simulink model "BidirectionalConverterBuckBoost"  (R2024a)
settings: Solver=VariableStepAuto  StartTime=0.0  StopTime=0.5  MaxStep=1e-6  RelTol=1e-3
undefined symbols (not defined in the file or in its folder): Ion, Lithium
libraries: spsSeriesRLCBranchLib x7, spsCurrentMeasurementLib x3, spsMosfetLib x2, spsVoltageMeasurementLib x2, spsBatteryLib x1, spsPVArrayLib x1, spsPWMGeneratorDCDCLib x1, SignalEditorBlockLib x1, sps_lib x1
settings Model: Creator=Owner  LastModifiedBy=Akbar
settings SolverCC: AlgebraicLoopSolver=TrustRegion
settings DebuggingCC: UnconnectedInputMsg=warning  UnconnectedOutputMsg=warning  UnconnectedLineMsg=warning
settings ModelReferenceCC: EnableRefExpFcnMdlSchedulingChecks=on
settings RTWCC: GPUComputeCapability=3.5

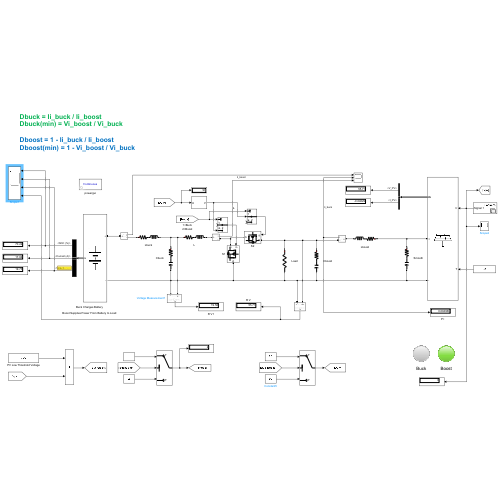
[thumbnail: Simulink's stored preview of the top-level diagram]
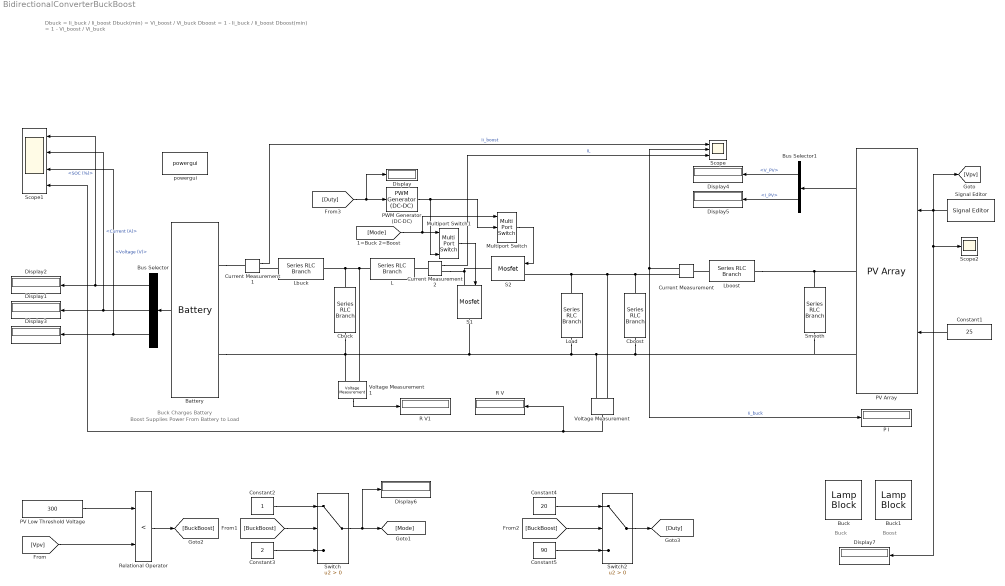
== system BidirectionalConverterBuckBoost ==
  note: Buck
  note: Buck Charges Battery
  note: Dbuck = Ii_buck / Ii_boost
      | Dbuck(min) = Vi_boost / Vi_buck
      |
      | Dboost = 1 - Ii_buck / Ii_boost
      | Dboost(min) = 1 - Vi_boost / Vi_buck
  note: Boost Supplies Power From Battery to Load
  note: Boost
  Battery : spsBatteryLib/Battery  BatType=Lithium-Ion  ShowTempParam=off  ThermalPreset=no  ShowAgeParam=off  NomV=25  NomQ=0.5  SOC=70  Batt_Tr=1  PresetModel=on  MaxQ=0.5  MinV=18.75  FullV=29.0997  Dis_rate=0.21739  R=0.5  Normal_OP=0.45217  expZone="[27.0096    0.0245652]"  current=[6.5 13 32.5]  Units=Time  Tci=20  NomT=20  T2=-30  MaxQ2=4.8  FullV2=7.1  Normal_OP2=5.655  expZone2="[6.58           1]"  Rca=0.6  ti=2000  Dp=0  Neq0=0  Tsim=1e6  Ta1=25  Qeol=5.4*0.9  Reol=0.013333*1.2  Char_age=[2.3478, 3]  Dis_age=[2.3478, 10]  N1=1500  N2=10500  N3=1000  N4=1400  Ta2=45  N5=950
  Buck : LampBlock  LabelPosition=Hide
  Buck1 : LampBlock  LabelPosition=Hide
  Bus Selector : BusSelector  OutputSignals=SOC (%),Current (A),Voltage (V)
  Bus Selector1 : BusSelector  OutputSignals=V_PV,I_PV
  Cboost : spsSeriesRLCBranchLib/Series RLC Branch  LConnTagsString=__new0  RConnTagsString=__new0  BranchType=RC  Resistance=0.1  Inductance=1e-3  SetiL0=off  InitialCurrent=0  Capacitance=1000e-6  Setx0=off  InitialVoltage=0  Measurements=None
  Cbuck : spsSeriesRLCBranchLib/Series RLC Branch  LConnTagsString=__new0  RConnTagsString=__new0  BranchType=RC  Resistance=0.1  Inductance=1e-3  SetiL0=off  InitialCurrent=0  Capacitance=1000e-6  Setx0=off  InitialVoltage=0  Measurements=None
  Constant1 : Constant  Value=25
  Constant2 : Constant
  Constant3 : Constant  Value=2
  Constant4 : Constant  Value=20
  Constant5 : Constant  Value=90
  Current Measurement : spsCurrentMeasurementLib/Current Measurement  PhasorSimulation=off  OutputType=Complex  PSBequivalent=0
  Current Measurement1 : spsCurrentMeasurementLib/Current Measurement  PhasorSimulation=off  OutputType=Complex  PSBequivalent=0
  Current Measurement2 : spsCurrentMeasurementLib/Current Measurement  PhasorSimulation=off  OutputType=Complex  PSBequivalent=0
  Display{,1..7} (8 alike) : Display
  L : spsSeriesRLCBranchLib/Series RLC Branch  LConnTagsString=__new0  RConnTagsString=__new0  BranchType=RL  Resistance=1  Inductance=3e-3  SetiL0=off  InitialCurrent=0  Capacitance=1e-6  Setx0=off  InitialVoltage=0  Measurements=None
  Lboost : spsSeriesRLCBranchLib/Series RLC Branch  LConnTagsString=__new0  RConnTagsString=__new0  BranchType=RL  Resistance=0.05  Inductance=150e-6  SetiL0=off  InitialCurrent=0  Capacitance=1000e-6  Setx0=off  InitialVoltage=0  Measurements=None
  Lbuck : spsSeriesRLCBranchLib/Series RLC Branch  LConnTagsString=__new0  RConnTagsString=__new0  BranchType=RL  Resistance=0.01  Inductance=50e-6  SetiL0=off  InitialCurrent=0  Capacitance=1000e-6  Setx0=off  InitialVoltage=0  Measurements=None
  Load : spsSeriesRLCBranchLib/Series RLC Branch  LConnTagsString=__new0  RConnTagsString=__new0  BranchType=R  Resistance=1000  Inductance=0  SetiL0=off  InitialCurrent=0  Capacitance=1000e-6  Setx0=off  InitialVoltage=0  Measurements=Branch voltage and current
  Multiport Switch : MultiPortSwitch  Inputs=2  SaturateOnIntegerOverflow=off  InputSameDT=off
  Multiport Switch1 : MultiPortSwitch  Inputs=2  SaturateOnIntegerOverflow=off  InputSameDT=off
  P I : Display
  PV Array : spsPVArrayLib/PV Array  Npar=40  Nser=2  PlotType=array @ 1000 W/m2 & specified temperatures  S_vec="[ 1000  500  100 ]"  Temp_C_vec="[ 45 25  ]"  ModuleName=User-defined  PlotWhenSelected=off  Pm=264.6  Ncell=60  Voc=44  Isc=7.84  Vm=36  Im=7.35  beta_Voc_pc=-0.36099  alpha_Isc_pc=0.102  beta_Voc=-0.15884  alpha_Isc=0.0079968  IL=7.9576  I0=2.9413e-10  nI=1.1899  Rsh=172.5073  Rs=0.34546  RobustModel=off  RobustCellTemperature=313.3991  BAL=on  Tc=1e-6  Tfilter=5e-5
  PV Low Threshold Voltage : Constant  Value=300
  PWM Generator (DC-DC) : spsPWMGeneratorDCDCLib/PWM Generator (DC-DC)  Fsw=30e3  Ts=0
  R V : Display
  R V1 : Display
  Relational Operator : RelationalOperator  Operator=<  OutDataTypeStr=boolean  RndMeth=Simplest  InputSameDT=off
  S1 : spsMosfetLib/Mosfet  Ron=0.1  Lon=0  Rd=0.01  Vfd=0  IC=0  Rs=1e5  Cs=inf  Measurements=off
  S2 : spsMosfetLib/Mosfet  Ron=0.1  Lon=0  Rd=0.01  Vfd=0  IC=0  Rs=1e5  Cs=inf  Measurements=off
  Scope : Scope  NumInputPorts=3
  Scope1 : Scope  NumInputPorts=4
  Scope2 : Scope
  Signal Editor : SignalEditorBlockLib/Signal Editor  FileName=C:\Users\Akbar\Cloud-Drive_maa32ocd@bolton.ac.uk\Hobby Projects\GitHub Repos\Matlab-Simulink\Renewable Energy\Bidirectional PV Battery Charging\RampUpDown.mat  ActiveScenario=Scenario  ActiveSignal=Signal 1  IsBus=off  OutputBusObjectStr=Bus: BusObject  SampleTime=0  ZeroCross=off  OutputAfterFinalValue=Setting to zero  Unit=inherit  PreserveSignalName=on  ApplySigPropsToAllScenarios=on  ApplySigPropsToAllSignals=off
  Smooth : spsSeriesRLCBranchLib/Series RLC Branch  LConnTagsString=__new0  RConnTagsString=__new0  BranchType=RC  Resistance=0.1  Inductance=1e-3  SetiL0=off  InitialCurrent=0  Capacitance=100e-5  Setx0=off  InitialVoltage=0  Measurements=None
  Switch : Switch  Criteria=u2 > Threshold  SaturateOnIntegerOverflow=off  InputSameDT=off
  Switch2 : Switch  Criteria=u2 > Threshold  SaturateOnIntegerOverflow=off  InputSameDT=off
  Voltage Measurement : spsVoltageMeasurementLib/Voltage Measurement  PhasorSimulation=off  OutputType=Complex  PSBequivalent=0
  Voltage Measurement1 : spsVoltageMeasurementLib/Voltage Measurement  PhasorSimulation=off  OutputType=Complex  PSBequivalent=0
  powergui : sps_lib/powergui  Priority=1  SimulationMode=Continuous  SampleTime=50e-6  frequency=60  Iterations=50  frequencyindice=0  Pbase=100e6  ErrMax=1e-4  UnitsV=kV  UnitsW=MW  buscounter=0  FunctionMessages=off  echomessages=off  EnableUseOfTLC=off  CurrentSourceSwitches=off  DisableSnubberDevices=off  DisableRonSwitches=off  DisableVfSwitches=off  DisplayEquations=off  AutomaticDiscreteSolvers=off  SolverType=Tustin/Backward Euler (TBE)  Interpol=off  ExternalGateDelay=off  methode=off  Ts=100  x0status=blocks  SPID=on  SwTol=0  HookPort=off  NonlinearTolerance=1e-4  nMaxIteration=100  ContinueOnMaxIteration=off  RestoreLinks=warning  ResistiveCurrentMeasurement=off  Frange=[0:2:500]  Ylog=off  Xlog=on  ShowGrid=off  save=off  variable=ZData  structure=0  ZoomFFT=off  StartTime=0.0  cycles=1  DisplayStyle=1  fundamental=60  FreqAxis=off  MaxFrequency=1000  frequencyindicesteady=1  RmsSteady=1  display=off
  wires:
  Multiport Switch/1 -> S2/1
  Multiport Switch1/1 -> S1/1
  [Mode] -> Multiport Switch/1, Multiport Switch1/1
  PWM Generator (DC-DC)/1 -> Multiport Switch1/3, Multiport Switch/2
  Current Measurement/1 -> P I/1, Scope/2  "Ii_buck"
  Current Measurement1/1 -> Scope/1  "Ii_boost"
  Current Measurement2/1 -> Scope/3  "IL"
  Battery/1 -> Bus Selector/1
  Bus Selector/1 -> Scope1/1, Display2/1  "<SOC (%)>"
  Bus Selector/2 -> Scope1/2, Display1/1  "<Current (A)>"
  Bus Selector/3 -> Scope1/3, Display3/1  "<Voltage (V)>"
  Constant1/1 -> PV Array/2
  PV Array/1 -> Bus Selector1/1
  Bus Selector1/1 -> Display4/1  "<V_PV>"
  Bus Selector1/2 -> Display5/1  "<I_PV>"
  Voltage Measurement/1 -> Scope1/4, R V/1
  Voltage Measurement1/1 -> R V1/1
  [Duty] -> Display/1, PWM Generator (DC-DC)/1
  PV Low Threshold Voltage/1 -> Relational Operator/1
  Constant2/1 -> Switch/1
  Constant3/1 -> Switch/3
  [Vpv] -> Relational Operator/2
  Switch/1 -> Display6/1, [Mode]
  Signal Editor/1 -> [Vpv], Display7/1, Scope2/1, PV Array/1
  Relational Operator/1 -> [BuckBoost]
  [BuckBoost] -> Switch/2
  [BuckBoost] -> Switch2/2
  Switch2/1 -> [Duty]
  Constant5/1 -> Switch2/3
  Constant4/1 -> Switch2/1
  connections:
  Current Measurement/RConn1 -- Voltage Measurement/LConn1 -- Load/LConn1 -- S2/LConn1 -- Cboost/LConn1
  S2/RConn1 -- Current Measurement2/RConn1 -- S1/LConn1
  Cbuck/RConn1 -- Voltage Measurement/LConn2 -- Smooth/RConn1 -- PV Array/RConn2 -- Cboost/RConn1 -- Load/RConn1 -- S1/RConn1 -- Voltage Measurement1/LConn2 -- Battery/LConn2
  Battery/LConn1 -- Current Measurement1/LConn1
  L/LConn1 -- Voltage Measurement1/LConn1 -- Cbuck/LConn1 -- Lbuck/RConn1
  Current Measurement2/LConn1 -- L/RConn1
  Lboost/RConn1 -- Current Measurement/LConn1
  Lbuck/LConn1 -- Current Measurement1/RConn1
  PV Array/RConn1 -- Smooth/LConn1 -- Lboost/LConn1
